simulink model "sl_flex"  (Simulink 7.7)
settings: Solver=ode45  StartTime=0.0  StopTime=4  RelTol=1e-3
PreLoadFcn:
  | twolink
libraries: roblocks x2
settings Model: Creator=pic  LastModifiedBy=corkep  ExtModeTrigMode=oneshot  ExtModeArmWhenConnect=off
settings DataIOCC: LimitDataPoints=off  ReturnWorkspaceOutputs=on
settings OptimizationCC: BlockReduction=off  BooleanDataType=off  InitFltsAndDblsToZero=on
settings DebuggingCC: SaveWithParameterizedLinksMsg=none  SignalResolutionControl=TryResolveAllWithWarning  SolverPrmCheckMsg=none  MultiTaskDSMMsg=warning  MultiTaskCondExecSysMsg=none  StrictBusMsg=None
settings HardwareCC: TargetUnknown=on
settings RTWCC: IncludeERTFirstTime=on
settings GRTTargetCC: ModelReferenceCompliant=off  CompOptLevelCompliant=off  MatFileLogging=off

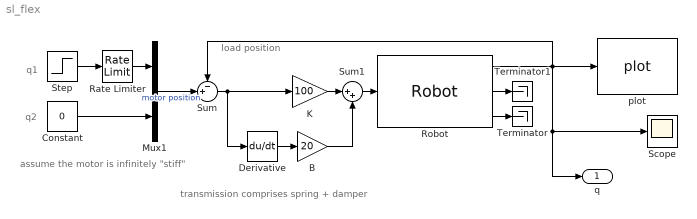
== system sl_flex ==
  note: load position
  note: transmission comprises
      | spring + damper
  note: assume the motor
      | is infinitely "stiff"
  note: q1
  note: q2
  B : Gain  Gain=20  SaturateOnIntegerOverflow=on  OutDataTypeStr=Inherit: Same as input  ParamDataTypeStr=Inherit: Same as input
  Constant : Constant  Value=0
  Derivative : Derivative
  K : Gain  Gain=100  SaturateOnIntegerOverflow=on  OutDataTypeStr=Inherit: Same as input  ParamDataTypeStr=Inherit: Same as input
  Mux1 : Mux  Inputs=2
  Rate Limiter : RateLimiter  RisingSlewLimit=50  FallingSlewLimit=-50
  Robot : roblocks/Dynamics/Robot  SystemSampleTime=-1  robot=twolink  q0=[0 0]
  Scope : Scope
      settings: YMin=-0.5  YMax=1.5
  Step : Step  SampleTime=0
  Sum : Sum  Inputs=-+|  SaturateOnIntegerOverflow=on  InputSameDT=on  OutDataTypeStr=Inherit: Same as first input
  Sum1 : Sum  Inputs=|++  SaturateOnIntegerOverflow=on  InputSameDT=on  OutDataTypeStr=Inherit: Same as first input
  Terminator : Terminator
  Terminator1 : Terminator
  plot : roblocks/Robot Graphics/plot  SystemSampleTime=-1  robot=twolink
  q : Outport
  wires:
  Constant/1 -> Mux1/2
  Step/1 -> Rate Limiter/1
  Rate Limiter/1 -> Mux1/1
  Sum/1 -> K/1, Derivative/1
  Robot/1 -> Sum/1, plot/1, Scope/1, q/1
  Sum1/1 -> Robot/1
  K/1 -> Sum1/1
  B/1 -> Sum1/2
  Derivative/1 -> B/1
  Mux1/1 -> Sum/2  "motor position"
  Robot/3 -> Terminator/1
  Robot/2 -> Terminator1/1
